simulink model "serialArduino"  (R2023b)
settings: Solver=VariableStepAuto  StartTime=0.0  StopTime=inf  RelTol=1e-3
undefined symbols (not defined in the file): LF
libraries: instrumentseriallib x3, etargetslib x1
settings Model: Creator=Bramantio  LastModifiedBy=Bramantio
settings OptimizationCC: ReuseModelBlockBuffer=off

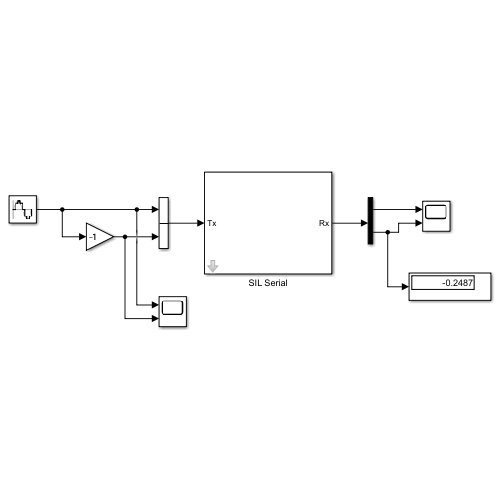
[thumbnail: Simulink's stored preview of the top-level diagram]
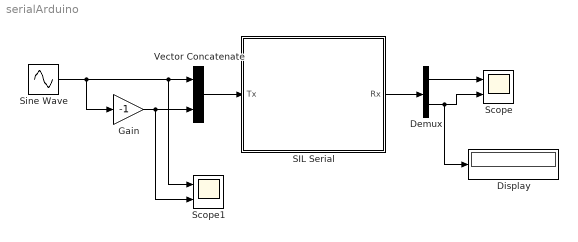
== system serialArduino ==
  Demux : Demux  Outputs=2
  Display : Display
  Gain : Gain  Gain=-1
  SIL Serial : Subsystem  mask{comport=COM11, data_size=2, sample_time=0.5, baud_rate=115200}
      mask prompts: comport "Serial Port (ex. "COM3")"; data_size "Data Size"; sample_time "Sample Time"; baud_rate "Baud Rate"
  Scope : Scope  NumInputPorts=2
  Scope1 : Scope  NumInputPorts=2
  Sine Wave : Sin  Frequency=2*pi*0.005  SampleTime=0.5
  Vector Concatenate : Concatenate
  wires:
  Gain/1 -> Scope1/2, Vector Concatenate/2
  Sine Wave/1 -> Scope1/1, Vector Concatenate/1, Gain/1
  Vector Concatenate/1 -> SIL Serial/1(Tx)
  SIL Serial/1(Rx) -> Demux/1
  Demux/1 -> Scope/1
  Demux/2 -> Display/1, Scope/2

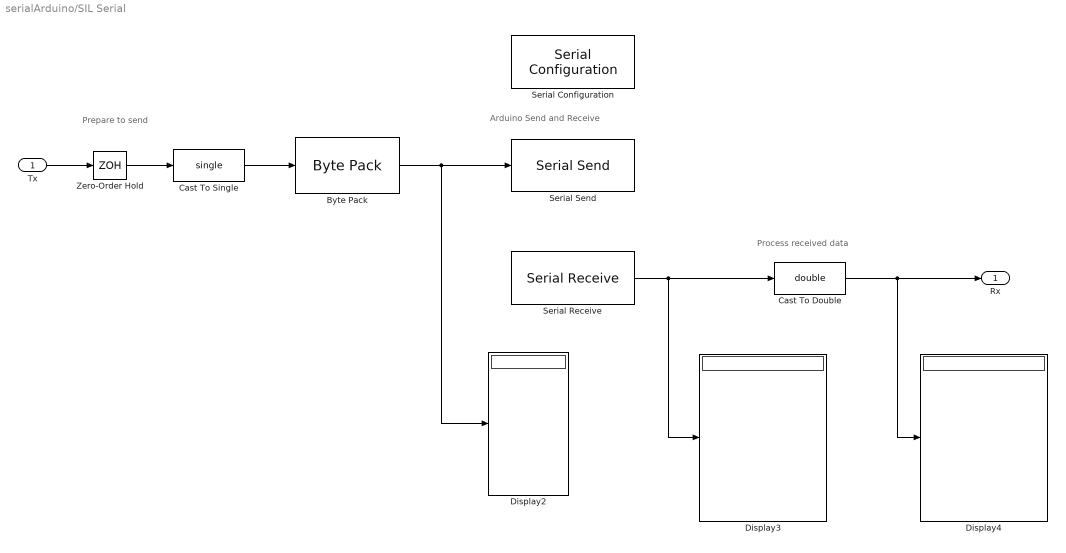
== system serialArduino/SIL Serial ==
  note: Prepare to send
  note: Arduino Send and Receive
  note: Process received data
  Tx : Inport
  Byte Pack : etargetslib/Byte Pack  datatypes={'single'}  byteAlign=4
  Cast To Double : DataTypeConversion  OutDataTypeStr=double  SaturateOnIntegerOverflow=off  RndMeth=Floor
  Cast To Single : DataTypeConversion  OutDataTypeStr=single  SaturateOnIntegerOverflow=off  RndMeth=Floor
  Display2 : Display
      settings: Format=hex (Stored Integer)
  Display3 : Display
  Display4 : Display
  Serial Configuration : instrumentseriallib/Serial Configuration  Priority=-200000  PortSel=comport  Port=comport  ComPort=comport  BaudRate=baud_rate  DataBits=8  Parity=none  StopBits=1  ByteOrder=little-endian  FlowControl=none  Timeout=10  SimulateUsing=Interpreted execution  BlockInModel=on  aMode=1
  Serial Receive : instrumentseriallib/Serial Receive  Priority=1  PortSel=comport  Port=comport  ComPort=comport  DataType=single  SaveDataType=uint8  ToggleHeader=on  Header=[ 65 ]  ToggleTerminator=on  Terminator=LF ('\n')  CustomTerminator=[]  InputFormat=Column major  ToggleDataSize=on  DataSize=[1 data_size]  EnableBlockingMode=on  ActionDataUnavailable=Output last received value  ActionWhenDataUnavailable=Output last received value  CustomValue=0  SampleTime=sample_time  SimulateUsing=Interpreted execution  BlockInModel=on  aMode=1
  Serial Send : instrumentseriallib/Serial Send  Priority=1  PortSel=comport  Port=comport  ComPort=comport  Header=[]  Terminator=LF ('\n')  CustomTerminator=[]  EnableBlockingMode=on  SimulateUsing=Interpreted execution  BlockInModel=on  aMode=1
  Zero-Order Hold : ZeroOrderHold  SampleTime=sample_time
  Rx : Outport
  wires:
  Tx/1 -> Zero-Order Hold/1
  Serial Receive/1 -> Display3/1, Cast To Double/1
  Zero-Order Hold/1 -> Cast To Single/1
  Byte Pack/1 -> Display2/1, Serial Send/1
  Cast To Double/1 -> Display4/1, Rx/1
  Cast To Single/1 -> Byte Pack/1
